simulink model "sl_ztorqueGravComp"  (R2014a)
settings: Solver=ode45  StartTime=0.0  StopTime=5  RelTol=1e-3
values from neighbouring files (symbols this model uses):
  q_in = [ 0 0 0 0 0 0]'    [Project3_Dockter.m]    (also in Project3sampleCode.m)
libraries: roblocks x3
settings Model: ExtModeTrigMode=oneshot  ExtModeArmWhenConnect=off  Creator=pic  LastModifiedBy=MRDLAB
settings DataIOCC: LimitDataPoints=off  SignalLoggingSaveFormat=ModelDataLogs  SignalLogging=off  ReturnWorkspaceOutputs=on
settings OptimizationCC: BlockReduction=off  BooleanDataType=off  ExpressionDepthLimit=2147483647  InitFltsAndDblsToZero=on
settings DebuggingCC: SaveWithParameterizedLinksMsg=none  UnderspecifiedInitializationDetection=Classic  SignalResolutionControl=TryResolveAllWithWarning  SolverPrmCheckMsg=none  MultiTaskDSMMsg=warning  MultiTaskCondExecSysMsg=none  FcnCallInpInsideContextMsg=UseLocalSettings  StateNameClashWarn=warning
settings HardwareCC: TargetUnknown=on
settings RTWCC: IncludeERTFirstTime=on
settings GRTTargetCC: ModelReferenceCompliant=off  ParMdlRefBuildCompliant=off  CompOptLevelCompliant=off  CombineOutputUpdateFcns=off  MatFileLogging=off  GRTInterface=on

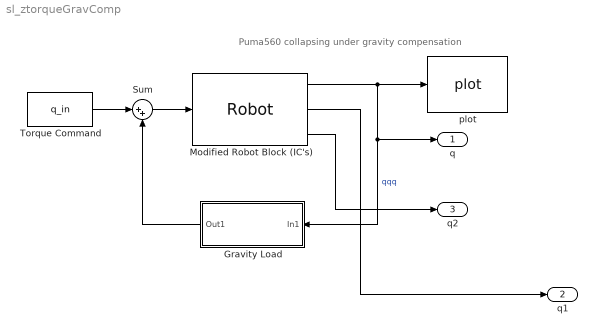
== system sl_ztorqueGravComp ==
  note: Puma560 collapsing under gravity compensation
  "Gravity Load " : Subsystem
  Modified Robot Block (IC's) : roblocks/Dynamics/Robot  robot=myRobot  q0=q0
      link override Integrator: InitialCondition=qd0
  Sum : Sum  Inputs=|++
  Torque Command : Constant  Value=q_in
  plot : roblocks/Robot Graphics/plot  robot=p560  fps=25  holdplot=on
  q : Outport
  q1 : Outport  Port=2
  q2 : Outport  Port=3
  wires:
  Torque Command/1 -> Sum/1
  Modified Robot Block (IC's)/1 -> plot/1, "Gravity Load "/1(In1), q/1  "qqq"
  Sum/1 -> Modified Robot Block (IC's)/1
  "Gravity Load "/1(Out1) -> Sum/2
  Modified Robot Block (IC's)/3 -> q2/1
  Modified Robot Block (IC's)/2 -> q1/1

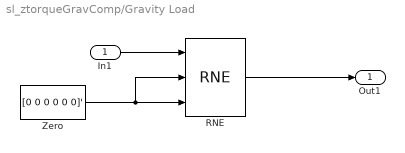
== system sl_ztorqueGravComp/Gravity Load  ==
  In1 : Inport
  RNE : roblocks/Dynamics/RNE  robot=myRobot  grav=[0 0 9.81]
  Zero : Constant  Value=[0 0 0 0 0 0]'
  Out1 : Outport
  wires:
  RNE/1 -> Out1/1
  Zero/1 -> RNE/3, RNE/2
  In1/1 -> RNE/1
